simulink model "gm_sampleModel1687_sub_sub"  (R2023a)
settings: Solver=VariableStepAuto  StartTime=0.0  StopTime=10.0  RelTol=1e-3
libraries: hdlsllib x5, simulink x2
settings Model: Creator=user1  LastModifiedBy=user1
settings OptimizationCC: BlockReduction=off  ConditionallyExecuteInputs=off
settings DebuggingCC: InheritedTsInSrcMsg=none

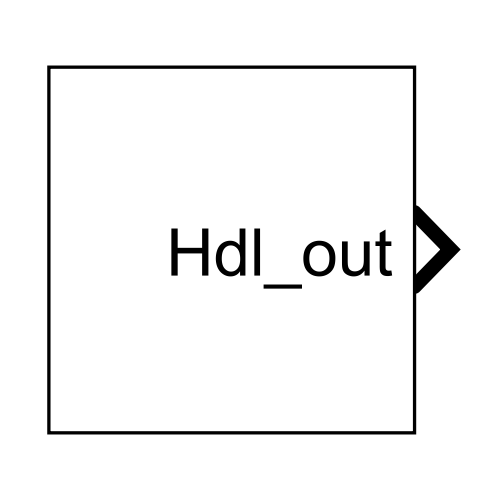
[thumbnail: Simulink's stored preview of the top-level diagram]
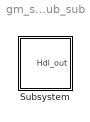
== system gm_sampleModel1687_sub_sub ==
  Subsystem : Subsystem

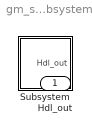
== system gm_sampleModel1687_sub_sub/Subsystem ==
  Subsystem : Subsystem
  Hdl_out : Outport  OutDataTypeStr=uint8

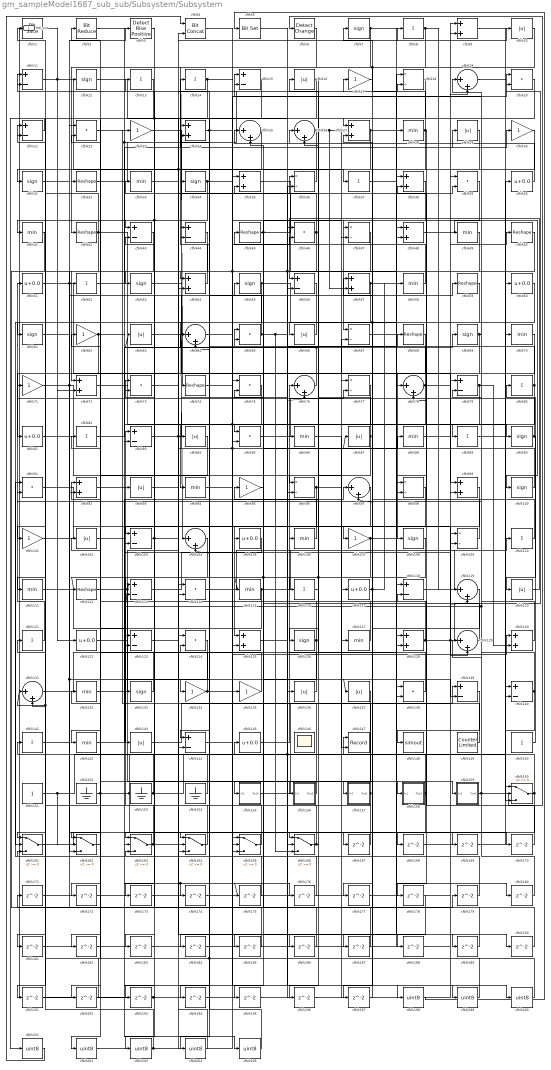
== system gm_sampleModel1687_sub_sub/Subsystem/Subsystem ==
  cfblk1 : hdlsllib/Logic and Bit Operations/Bit Slice  lidx=7  ridx=0
  cfblk{10,16,29,63,66,84,87,93,102,120,136..137,143} (13 alike) : Abs  OutDataTypeStr=uint8  SaturateOnIntegerOverflow=off
  cfblk{7,12,31,34,53,55,61,69,90,100,108,126,133} (13 alike) : Signum
  cfblk{17,23,30,62,71,95,101,107,134..135} (10 alike) : Gain  OutDataTypeStr=uint8
  cfblk{11,15,21,43..44,56,79,83,103,113,118,123,139..140,144} (15 alike) : Sum  Inputs=+-  OutDataTypeStr=uint8
  cfblk{19,25..26,64,76,78,97,104,119,129,131} (11 alike) : Sum  Inputs=|++  OutDataTypeStr=uint8
  cfblk{40,51,60,81,105,117,122,145} (8 alike) : Bias  Bias=0.0  SaturateOnIntegerOverflow=off
  cfblk{28,33,41,49,58,70,86,88,94,106,111,115,127,132,142} (15 alike) : MinMax  OutDataTypeStr=uint8
  cfblk{18,36,47,67,77,96,98,109} (8 alike) : Product  Inputs=*/  OutDataTypeStr=uint8  RndMeth=Zero  SaturateOnIntegerOverflow=on
  cfblk{8,13..14,37,52,80,82,89,110,116,121,141} (12 alike) : Sum  Inputs=+  OutDataTypeStr=uint8
  cfblk{32,42,45,50,59,68,74,112} (8 alike) : Reshape
  cfblk{20,22,39,46,65,73,75,85,91,114,124,138} (12 alike) : DotProduct  OutDataTypeStr=uint8
  cfblk{9,24,27,35,38,48,54,57,72,92,99,125,128,130} (14 alike) : Sum  OutDataTypeStr=uint8
  cfblk146 : Scope
      settings: Floating=on
  cfblk147 : Record  FileSettingsInternal="{\"entries\":[{\"content\":{\"excelSettings\":{\"content\":{},\"type\":\"Streamout.ExcelSettings\"}},\"type\":\"Streamout.FileSettingStorage\",\"uuid\":\"\"}],\"packageUris\":[\"http:\\/\\/schema.mathworks.com\\/mf0\\/streamout_blocks\\/R2020a\"],\"version\":\"1.0\"}"  Layout=[1 1]  SignalsInternal="{\"entries\":[{\"content\":{\"signals\":[{\"content\":{\"blockPath\":[],\"dimensions\":[1],\"domain\":\"\",\"lineColor\":\"#a2142f\",\"plots\":[1],\"port\":1,\"signalID\":35156,\"signalName\":\"cfblk158\"},\"type\":\"RecordBlkView.Signal\",\"uuid\":\"\"},{\"content\":{\"blockPath\":[],\"dimensions\":[1],\"domain\":\"\",\"lineColor\":\"#139fff\",\"plots\":[1],\"port\":2,\"signalID\":35159,\"signalName\":\"cfblk71\"},\"type\":\"RecordBlkView.Signal\",\"uuid\":\"\"}]},\"type\":\"RecordBlkView.InputSignals\",\"uuid\":\"\"}],\"packageUris\":[\"http:\\/\\/schema.mathworks.com\\/mf0\\/streamout_blocks\\/R2020a\"],\"version\":\"1.0\"}"  VisualizationBindings="{\"xyplotplugin\":{\"info\":[{\"series\":[{\"bindingParametersList\":[{\"parameter\":\"X-Axis\",\"signalID\":35156,\"signalName\":\"cfblk158\"},{\"parameter\":\"Y-Axis\",\"signalID\":35159,\"signalName\":\"cfblk71\"}],\"seriesID\":19763}],\"subplotID\":1}]}}"  CompatibilityTag=XY  st=-1
  cfblk148 : ToWorkspace  VariableName=simout  SaveFormat=Timeseries  SampleTime=-1
  cfblk149 : hdlsllib/Sources/Counter Limited  uplimit=7  tsamp=-1
  cfblk150 : Constant  OutDataTypeStr=uint8  SampleTime=-1
  cfblk151 : Constant  OutDataTypeStr=uint8  SampleTime=-1
  cfblk152 : Ground
  cfblk153 : Ground
  cfblk154 : Ground
  cfblk155 : Subsystem
      settings: LibrarySourceBlock=|
      | hdlsllib/Ports &
      | Subsystems/Subsystem
  cfblk156 : Subsystem
      settings: LibrarySourceBlock=|
      | hdlsllib/Ports &
      | Subsystems/Subsystem
  cfblk157 : Subsystem
      settings: LibrarySourceBlock=|
      | hdlsllib/Ports &
      | Subsystems/Subsystem
  cfblk158 : Subsystem
      settings: LibrarySourceBlock=|
      | hdlsllib/Ports &
      | Subsystems/Subsystem
  cfblk159 : Subsystem
      settings: LibrarySourceBlock=|
      | hdlsllib/Ports &
      | Subsystems/Subsystem
  cfblk{160..166} (7 alike) : Switch  OutDataTypeStr=uint8  SaturateOnIntegerOverflow=off  InputSameDT=off
  cfblk{167..197} (31 alike) : Delay  SampleTime=1
  cfblk{198..205} (8 alike) : DataTypeConversion  OutDataTypeStr=uint8  SaturateOnIntegerOverflow=off  RndMeth=Floor
  cfblk2 : hdlsllib/Logic and Bit Operations/Bit Reduce  mode=AND
  cfblk3 : hdlsllib/Logic and Bit Operations/Detect Rise Positive  vinit=0  OutDataTypeStr=uint8
  cfblk4 : hdlsllib/Logic and Bit Operations/Bit Concat  numInputs=2
  cfblk5 : simulink/Logic and Bit Operations/Bit Set  iBit=0
      settings: LibrarySourceBlock=|
      | hdlsllib/Logic and Bit
      | Operations/Bit Set
  cfblk6 : simulink/Logic and Bit Operations/Detect Change  vinit=0  OutDataTypeStr=uint8
      settings: LibrarySourceBlock=|
      | hdlsllib/Logic and Bit
      | Operations/Detect
      | Change
  Hdl_out : Outport  OutDataTypeStr=uint8
  wires:
  cfblk60/1 -> cfblk197/1, cfblk104/1
  cfblk65/1 -> cfblk44/2, cfblk167/1, cfblk166/3
  cfblk105/1 -> cfblk83/1
  cfblk156/1(Out1) -> cfblk23/1
  cfblk82/1 -> cfblk69/1
  cfblk103/1 -> cfblk173/1, cfblk15/1
  cfblk121/1 -> cfblk51/1
  cfblk10/1 -> cfblk47/1, cfblk74/1
  cfblk124/1 -> cfblk203/1
  cfblk96/1 -> cfblk184/1, cfblk139/2
  cfblk48/1 -> cfblk100/1
  cfblk77/1 -> cfblk95/1
  cfblk120/1 -> cfblk56/1
  cfblk1/1 -> cfblk122/1
  cfblk165/1 -> cfblk93/1
  cfblk43/1 -> cfblk72/1
  cfblk32/1 -> cfblk17/1
  cfblk145/1 -> cfblk76/1
  cfblk157/1(Out1) -> cfblk44/1, cfblk145/1
  cfblk42/1 -> cfblk162/3, cfblk11/2, cfblk90/1
  cfblk49/1 -> cfblk194/1, cfblk165/3
  cfblk154/1 -> cfblk1/1
  cfblk23/1 -> cfblk108/1
  cfblk67/1 -> cfblk118/1
  cfblk81/1 -> cfblk96/1
  cfblk18/1 -> cfblk42/1
  cfblk34/1 -> cfblk30/1, cfblk183/1, cfblk181/1
  cfblk79/1 -> cfblk178/1, cfblk130/2
  cfblk75/1 -> cfblk94/1
  cfblk71/1 -> cfblk147/2, cfblk59/1
  cfblk112/1 -> cfblk88/1, cfblk158/1(In1)
  cfblk35/1 -> cfblk128/1
  cfblk54/1 -> cfblk14/1
  cfblk99/1 -> cfblk103/1
  cfblk128/1 -> cfblk82/1, cfblk119/2, cfblk20/1
  cfblk116/1 -> cfblk26/1
  cfblk88/1 -> cfblk49/1
  cfblk62/1 -> cfblk92/2, cfblk175/1, cfblk174/1
  cfblk94/1 -> cfblk20/2, cfblk87/1
  cfblk113/1 -> cfblk79/1
  cfblk38/1 -> cfblk115/1, cfblk155/1(In1)
  cfblk19/1 -> cfblk160/1
  cfblk36/1 -> cfblk31/1
  cfblk136/1 -> cfblk106/1
  cfblk12/1 -> cfblk136/1
  cfblk93/1 -> cfblk10/1
  cfblk46/1 -> cfblk111/1, cfblk13/1
  cfblk159/1(Out1) -> cfblk79/2, cfblk6/1
  cfblk160/1 -> cfblk193/1, cfblk21/1
  cfblk122/1 -> cfblk36/1
  cfblk115/1 -> cfblk162/1, cfblk9/1
  cfblk76/1 -> cfblk55/1, cfblk63/1
  cfblk155/1(Out1) -> cfblk139/1
  cfblk27/1 -> cfblk89/1, cfblk101/1
  cfblk97/1 -> cfblk125/1
  cfblk101/1 -> cfblk105/1
  cfblk104/1 -> cfblk142/1
  cfblk140/1 -> cfblk160/3, cfblk113/1, cfblk91/2
  cfblk74/1 -> cfblk39/2
  cfblk163/1 -> cfblk169/1, cfblk22/2
  cfblk151/1 -> cfblk162/2, cfblk76/2, cfblk40/1
  cfblk100/1 -> cfblk65/1
  cfblk3/1 -> cfblk53/1
  cfblk134/1 -> cfblk46/2, cfblk33/1
  cfblk44/1 -> cfblk54/1
  cfblk47/1 -> cfblk84/1, cfblk96/2
  cfblk51/1 -> cfblk114/1, cfblk137/1, cfblk163/2
  cfblk132/1 -> cfblk8/1
  cfblk144/1 -> cfblk130/1
  cfblk28/1 -> cfblk98/1, cfblk7/1, cfblk191/1, cfblk144/2
  cfblk131/1 -> cfblk48/2
  cfblk6/1 -> cfblk43/1
  cfblk162/1 -> cfblk92/1
  cfblk111/1 -> cfblk143/1
  cfblk114/1 -> cfblk70/1
  cfblk127/1 -> cfblk16/1
  cfblk110/1 -> cfblk45/1
  cfblk7/1 -> cfblk190/1, cfblk32/1
  cfblk108/1 -> cfblk126/1, cfblk112/1
  cfblk166/1 -> cfblk196/1, cfblk73/1
  cfblk107/1 -> cfblk189/1, cfblk123/1
  cfblk25/1 -> cfblk163/1
  cfblk109/1 -> cfblk38/2
  cfblk126/1 -> cfblk195/1, cfblk24/1
  cfblk17/1 -> cfblk107/1
  cfblk85/1 -> cfblk77/2
  cfblk142/1 -> cfblk97/1
  cfblk69/1 -> cfblk78/2, cfblk19/1
  cfblk138/1 -> cfblk86/1
  cfblk106/1 -> cfblk75/2
  cfblk20/1 -> cfblk133/1, cfblk161/1
  cfblk24/1 -> cfblk47/2, cfblk134/1
  cfblk164/1 -> cfblk121/1, cfblk131/1
  cfblk90/1 -> cfblk71/1, cfblk120/1
  cfblk73/1 -> cfblk156/1(In1)
  cfblk9/1 -> cfblk140/1
  cfblk39/1 -> cfblk67/1
  cfblk139/1 -> cfblk148/1
  cfblk64/1 -> cfblk109/2
  cfblk86/1 -> cfblk127/1
  cfblk5/1 -> cfblk199/1
  cfblk129/1 -> cfblk35/2
  cfblk78/1 -> cfblk113/2, cfblk50/1, cfblk34/1
  cfblk8/1 -> cfblk119/1, cfblk27/1
  cfblk68/1 -> cfblk81/1
  cfblk40/1 -> cfblk25/1
  cfblk45/1 -> cfblk85/1, cfblk19/2
  cfblk59/1 -> cfblk116/1
  cfblk130/1 -> cfblk15/2
  cfblk63/1 -> cfblk46/1
  cfblk95/1 -> cfblk25/2
  cfblk153/1 -> cfblk56/2, cfblk21/2
  cfblk50/1 -> cfblk83/2
  cfblk66/1 -> cfblk61/1
  cfblk135/1 -> cfblk62/1
  cfblk53/1 -> cfblk99/1
  cfblk61/1 -> cfblk3/1
  cfblk56/1 -> cfblk66/1
  cfblk152/1 -> cfblk132/1, cfblk164/3, cfblk117/1
  cfblk117/1 -> cfblk58/1, cfblk97/2
  cfblk87/1 -> cfblk166/1, cfblk64/1
  cfblk133/1 -> cfblk102/1
  cfblk11/1 -> cfblk72/2, cfblk37/1
  cfblk55/1 -> cfblk138/2, cfblk161/2
  cfblk102/1 -> cfblk123/2
  cfblk119/1 -> cfblk157/1(In1)
  cfblk143/1 -> cfblk28/1
  cfblk72/1 -> cfblk98/2, cfblk135/1
  cfblk83/1 -> cfblk185/1, cfblk68/1
  cfblk149/1 -> cfblk57/1
  cfblk58/1 -> cfblk26/2
  cfblk80/1 -> cfblk11/1, cfblk103/2
  cfblk13/1 -> cfblk52/1
  cfblk118/1 -> cfblk110/1
  cfblk26/1 -> cfblk54/2, cfblk78/1, cfblk57/2
  cfblk14/1 -> cfblk41/1, cfblk159/1(In1)
  cfblk161/1 -> cfblk164/1
  cfblk52/1 -> cfblk29/1
  cfblk22/1 -> cfblk198/1, cfblk24/2
  cfblk15/1 -> cfblk114/2
  cfblk33/1 -> cfblk18/2
  cfblk16/1 -> cfblk186/1, cfblk144/1
  cfblk57/1 -> cfblk180/1, cfblk125/2
  cfblk31/1 -> cfblk12/1
  cfblk150/1 -> cfblk80/1
  cfblk37/1 -> cfblk138/1
  cfblk91/1 -> cfblk129/2
  cfblk89/1 -> cfblk60/1
  cfblk158/1(Out1) -> cfblk165/2, cfblk147/1
  cfblk167/1 -> cfblk75/1
  cfblk141/1 -> cfblk168/1
  cfblk168/1 -> cfblk140/2
  cfblk169/1 -> cfblk160/2
  cfblk125/1 -> cfblk170/1
  cfblk170/1 -> cfblk118/2
  cfblk171/1 -> cfblk164/2
  cfblk70/1 -> cfblk172/1
  cfblk172/1 -> cfblk48/1
  cfblk173/1 -> cfblk99/2
  cfblk174/1 -> cfblk18/1
  cfblk175/1 -> cfblk43/2
  cfblk92/1 -> cfblk176/1
  cfblk176/1 -> cfblk91/1
  cfblk98/1 -> cfblk177/1
  cfblk177/1 -> cfblk38/1
  cfblk41/1 -> cfblk179/1
  cfblk179/1 -> cfblk64/2
  cfblk180/1 -> cfblk129/1
  cfblk181/1 -> cfblk77/1
  cfblk30/1 -> cfblk182/1
  cfblk182/1 -> cfblk128/2
  cfblk183/1 -> cfblk166/2
  cfblk184/1 -> cfblk35/1
  cfblk185/1 -> cfblk73/2
  cfblk186/1 -> cfblk22/1
  cfblk29/1 -> cfblk187/1
  cfblk187/1 -> cfblk65/2
  cfblk123/1 -> cfblk188/1
  cfblk188/1 -> cfblk39/1
  cfblk189/1 -> cfblk163/3
  cfblk190/1 -> cfblk131/2
  cfblk191/1 -> cfblk165/1
  cfblk84/1 -> cfblk192/1
  cfblk192/1 -> cfblk161/3
  cfblk193/1 -> Hdl_out/1, cfblk67/2
  cfblk194/1 -> cfblk109/1
  cfblk195/1 -> cfblk36/2
  cfblk196/1 -> cfblk9/2
  cfblk197/1 -> cfblk27/2
  cfblk198/1 -> cfblk5/1
  cfblk199/1 -> cfblk104/2, cfblk171/1
  cfblk4/1 -> cfblk200/1
  cfblk200/1 -> cfblk2/1
  cfblk21/1 -> cfblk201/1
  cfblk201/1 -> cfblk4/1
  cfblk137/1 -> cfblk202/1
  cfblk202/1 -> cfblk4/2
  cfblk203/1 -> cfblk141/1, cfblk85/2
  cfblk178/1 -> cfblk204/1
  cfblk204/1 -> cfblk124/1
  cfblk2/1 -> cfblk205/1
  cfblk205/1 -> cfblk124/2

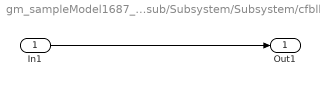
== system gm_sampleModel1687_sub_sub/Subsystem/Subsystem/cfblk155 ==
  In1 : Inport
  Out1 : Outport
  wires:
  In1/1 -> Out1/1

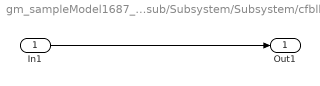
== system gm_sampleModel1687_sub_sub/Subsystem/Subsystem/cfblk156 ==
  In1 : Inport
  Out1 : Outport
  wires:
  In1/1 -> Out1/1

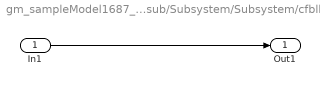
== system gm_sampleModel1687_sub_sub/Subsystem/Subsystem/cfblk157 ==
  In1 : Inport
  Out1 : Outport
  wires:
  In1/1 -> Out1/1

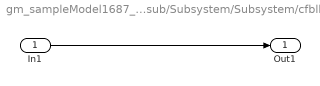
== system gm_sampleModel1687_sub_sub/Subsystem/Subsystem/cfblk158 ==
  In1 : Inport
  Out1 : Outport
  wires:
  In1/1 -> Out1/1

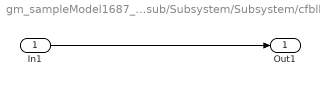
== system gm_sampleModel1687_sub_sub/Subsystem/Subsystem/cfblk159 ==
  In1 : Inport
  Out1 : Outport
  wires:
  In1/1 -> Out1/1
